simulink model "myExampleModel"  (R2026a)
settings: Solver=FixedStepDiscrete  StopTime=steps  FixedStep=1
model workspace (MAT data in the model file):
  net = dlnetwork
  net.any.Version = 6
  net.any.LayerGraph = nnet.cnn.LayerGraph
  net.any.LayerGraph.any.Version = 1
  net.any.LayerGraph.any.Layers(1) = nnet.cnn.layer.SequenceInputLayer
  net.any.LayerGraph.any.Layers(1).any.Version = 5
  net.any.LayerGraph.any.Layers(1).any.Name = 'sequenceinput'
  net.any.LayerGraph.any.Layers(1).any.InputSize = 5
  net.any.LayerGraph.any.Layers(1).any.Normalization.Version = 1
  net.any.LayerGraph.any.Layers(1).any.Normalization.Type = 'zscore'
  net.any.LayerGraph.any.Layers(1).any.Normalization.ImageSize = 5
  net.any.LayerGraph.any.Layers(1).any.Normalization.Mean = [0.711946004247; 0.753163225915; 0.731572433704; 0.711407042817; 0.753343332248]
  net.any.LayerGraph.any.Layers(1).any.Normalization.Std = [0.253594852887; 0.0795590152826; 0.271454001973; 0.250256363005; 0.0564169836974]
  net.any.LayerGraph.any.Layers(1).any.NormalizationDimension = 'auto'
  net.any.LayerGraph.any.Layers(1).any.MinLength = 1
  net.any.LayerGraph.any.Layers(1).any.SplitComplexInputs = 0
  net.any.LayerGraph.any.Layers(2) = nnet.cnn.layer.LSTMLayer
  net.any.LayerGraph.any.Layers(2).any.Version = 5
  net.any.LayerGraph.any.Layers(2).any.Name = 'lstm'
  net.any.LayerGraph.any.Layers(2).any.InputSize = 5
  net.any.LayerGraph.any.Layers(2).any.NumHiddenUnits = 32
  net.any.LayerGraph.any.Layers(2).any.ReturnSequence = 1
  net.any.LayerGraph.any.Layers(2).any.StateActivationFunction = 'tanh'
  net.any.LayerGraph.any.Layers(2).any.GateActivationFunction = 'sigmoid'
  net.any.LayerGraph.any.Layers(2).any.HasStateInputs = 0
  net.any.LayerGraph.any.Layers(2).any.HasStateOutputs = 0
  net.any.LayerGraph.any.Layers(2).any.InputWeights.Version = 2
  net.any.LayerGraph.any.Layers(2).any.InputWeights.Value = [0.158725649118 0.0836796313524 0.0394077338278 0.00389027385972 0.00940972659737 -0.159172236919 0.180239677429 0.0973209440708 -0.0486048273742 0.142829716206 0.0468379706144 -0.109037384391 ... (640 elements, 128x5)]
  net.any.LayerGraph.any.Layers(2).any.InputWeights.LearnRateFactor = 1
  net.any.LayerGraph.any.Layers(2).any.InputWeights.L2Factor = 1
  net.any.LayerGraph.any.Layers(2).any.InputWeights.Initializer.Version = 1
  net.any.LayerGraph.any.Layers(2).any.InputWeights.Initializer.Class = 'nnet.internal.cnn.layer.learnable.initializer.Glorot'
  net.any.LayerGraph.any.Layers(2).any.InputWeights.Initializer.ConstructorArguments = {2, 1}
  net.any.LayerGraph.any.Layers(2).any.RecurrentWeights.Version = 2
  net.any.LayerGraph.any.Layers(2).any.RecurrentWeights.Value = [-0.0278804842383 -0.025140536949 -0.0255219098181 -0.0234189406037 -0.0516594834626 -0.0393797829747 -0.0177398081869 -0.0392154678702 -0.105208314955 -0.100077986717 -0.0357415638864 0.0239775925875 ... (4096 elements, 128x32)]
  net.any.LayerGraph.any.Layers(2).any.RecurrentWeights.LearnRateFactor = 1
  net.any.LayerGraph.any.Layers(2).any.RecurrentWeights.L2Factor = 1
  net.any.LayerGraph.any.Layers(2).any.RecurrentWeights.Initializer.Version = 1
  net.any.LayerGraph.any.Layers(2).any.RecurrentWeights.Initializer.Class = 'nnet.internal.cnn.layer.learnable.initializer.Orthogonal'
  net.any.LayerGraph.any.Layers(2).any.RecurrentWeights.Initializer.ConstructorArguments = []
  net.any.LayerGraph.any.Layers(2).any.Bias.Version = 2
  net.any.LayerGraph.any.Layers(2).any.Bias.Value = [-0.0182774588466 0.0614794008434 0.0734638869762 -0.0580208562315 -0.0653121620417 0.113746903837 0.0700471177697 0.0615480169654 0.0146696139127 0.0178057868034 0.0246399398893 0.0890641435981 ... (128 elements, 128x1)]
  net.any.LayerGraph.any.Layers(2).any.Bias.LearnRateFactor = 1
  net.any.LayerGraph.any.Layers(2).any.Bias.L2Factor = 0
  net.any.LayerGraph.any.Layers(2).any.Bias.Initializer.Version = 1
  net.any.LayerGraph.any.Layers(2).any.Bias.Initializer.Class = 'nnet.internal.cnn.layer.learnable.initializer.UnitForgetGate'
  net.any.LayerGraph.any.Layers(2).any.Bias.Initializer.ConstructorArguments = {'LSTM'}
  net.any.LayerGraph.any.Layers(2).any.CellState.Value = [0; 0; 0; 0; 0; 0; 0; 0; 0; 0; 0; 0; 0; 0; 0; 0; 0; 0; 0; 0; 0; 0; 0; 0; 0; 0; 0; 0; 0; 0; 0; 0]
  net.any.LayerGraph.any.Layers(2).any.CellState.Remember = 1
  net.any.LayerGraph.any.Layers(2).any.HiddenState.Value = [0; 0; 0; 0; 0; 0; 0; 0; 0; 0; 0; 0; 0; 0; 0; 0; 0; 0; 0; 0; 0; 0; 0; 0; 0; 0; 0; 0; 0; 0; 0; 0]
  net.any.LayerGraph.any.Layers(2).any.HiddenState.Remember = 1
  net.any.LayerGraph.any.Layers(2).any.InitialCellState = [0; 0; 0; 0; 0; 0; 0; 0; 0; 0; 0; 0; 0; 0; 0; 0; 0; 0; 0; 0; 0; 0; 0; 0; 0; 0; 0; 0; 0; 0; 0; 0]
  net.any.LayerGraph.any.Layers(2).any.InitialHiddenState = [0; 0; 0; 0; 0; 0; 0; 0; 0; 0; 0; 0; 0; 0; 0; 0; 0; 0; 0; 0; 0; 0; 0; 0; 0; 0; 0; 0; 0; 0; 0; 0]
  net.any.LayerGraph.any.Layers(3) = nnet.cnn.layer.FullyConnectedLayer
  net.any.LayerGraph.any.Layers(3).any.Version = 5
  net.any.LayerGraph.any.Layers(3).any.Name = 'fc'
  net.any.LayerGraph.any.Layers(3).any.InputSize = []
  net.any.LayerGraph.any.Layers(3).any.OutputSize = 1
  net.any.LayerGraph.any.Layers(3).any.Weights.Version = 2
  net.any.LayerGraph.any.Layers(3).any.Weights.Value = [-0.0115323774517 -0.22575378418 0.0668845772743 0.308706641197 0.18884755671 0.224740937352 0.278032541275 0.305149555206 -0.0114221740514 -0.165821552277 -0.413473755121 -0.363296926022 -0.351468086243 0.283178627491 -0.0468922816217 -0.19526720047 0.115473456681 0.11662748456 -0.427064061165 0.384527653456 -0.253217667341 -0.318987667561 -0.351537317038 0.306988537312 -0.314961463213 0.122481673956 0.0571382455528 0.390641868114 0.372646659613 0.330578863621 -0.47236636281 0.24124994874]
  net.any.LayerGraph.any.Layers(3).any.Weights.LearnRateFactor = 1
  net.any.LayerGraph.any.Layers(3).any.Weights.L2Factor = 1
  net.any.LayerGraph.any.Layers(3).any.Weights.Initializer.Version = 1
  net.any.LayerGraph.any.Layers(3).any.Weights.Initializer.Class = 'nnet.internal.cnn.layer.learnable.initializer.Glorot'
  net.any.LayerGraph.any.Layers(3).any.Weights.Initializer.ConstructorArguments = {2, 1}
  net.any.LayerGraph.any.Layers(3).any.Bias.Version = 2
  net.any.LayerGraph.any.Layers(3).any.Bias.Value = -0.000715207715984
  net.any.LayerGraph.any.Layers(3).any.Bias.LearnRateFactor = 1
  net.any.LayerGraph.any.Layers(3).any.Bias.L2Factor = 0
  net.any.LayerGraph.any.Layers(3).any.Bias.Initializer.Version = 1
  net.any.LayerGraph.any.Layers(3).any.Bias.Initializer.Class = 'nnet.internal.cnn.layer.learnable.initializer.Zeros'
  net.any.LayerGraph.any.Layers(3).any.Bias.Initializer.ConstructorArguments = []
  net.any.LayerGraph.any.Layers(3).any.InputLearnables = {}
  net.any.LayerGraph.any.Layers(3).any.OutputLearnables = {}
  net.any.LayerGraph.any.Layers(3).any.OperationDimension = 'spatial-channel'
  net.any.LayerGraph.any.Layers(4) = nnet.cnn.layer.InverseNormalizationLayer
  net.any.LayerGraph.any.Layers(4).Name = 'inversenorm'
  net.any.LayerGraph.any.Layers(4).Normalization = 'zscore'
  net.any.LayerGraph.any.Layers(4).OperationDimension = 'channel'
  net.any.LayerGraph.any.Layers(4).Mean = 0.633833984011
  net.any.LayerGraph.any.Layers(4).StandardDeviation = 0.340294791967
  net.any.LayerGraph.any.Connections = table
  net.any.LayerGraph.any.Connections.data = {{'sequenceinput'; 'lstm'; 'fc'}, {'lstm'; 'fc'; 'inversenorm'}}
  net.any.LayerGraph.any.Connections.ndims = 2
  net.any.LayerGraph.any.Connections.nrows = 3
  net.any.LayerGraph.any.Connections.nvars = 2
  net.any.LayerGraph.any.Connections.varnames = {'Source', 'Destination'}
  net.any.LayerGraph.any.Connections.props.CustomProps = struct()
  net.any.LayerGraph.any.Connections.props.VariableCustomProps = struct()
  net.any.LayerGraph.any.Connections.props.versionSavedFrom = 5
  net.any.LayerGraph.any.Connections.props.minCompatibleVersion = 1
  net.any.LayerGraph.any.Connections.props.incompatibilityMsg = ''
  net.any.LayerGraph.any.Connections.props.VersionSavedFrom = 5
  net.any.LayerGraph.any.Connections.props.useVariableNamesOriginal = 0
  net.any.LayerGraph.any.Connections.props.useVariableNames2048 = 0
  net.any.LayerGraph.any.Connections.props.useDimensionNamesOriginal = 0
  net.any.LayerGraph.any.Connections.props.useDimensionNames2048 = 0
  net.any.LayerGraph.any.Connections.props.Description = ''
  net.any.LayerGraph.any.Connections.props.VariableNamesOriginal = {}
  net.any.LayerGraph.any.Connections.props.VariableNames2048 = {}
  net.any.LayerGraph.any.Connections.props.DimensionNames = {'Row', 'Variables'}
  net.any.LayerGraph.any.Connections.props.DimensionNamesOriginal = {}
  net.any.LayerGraph.any.Connections.props.DimensionNames2048 = {}
  net.any.LayerGraph.any.Connections.props.UserData = []
  net.any.LayerGraph.any.Connections.props.VariableDescriptions = {}
  net.any.LayerGraph.any.Connections.props.VariableUnits = {}
  net.any.LayerGraph.any.Connections.props.VariableContinuity = {}
  net.any.Initialized = 1
  net.any.SerializedQuantizationInfo.version = 1
  net.any.SerializedQuantizationInfo.data = containers.Map
  net.any.SerializedQuantizationInfo.data.serialization.keys = {}
  net.any.SerializedQuantizationInfo.data.serialization.values = {}
  net.any.SerializedQuantizationInfo.data.serialization.uniformity = 0
  net.any.SerializedQuantizationInfo.data.serialization.keyType = 'char'
  net.any.SerializedQuantizationInfo.data.serialization.valueType = 'any'
  net.any.ExampleInputs = {}
  net.any.OutputNames = {'inversenorm'}
  net.any.ExternalOutputNames = []
  net.any.ExternalInputNames = []
  net.any.RetainCustomInputNames = 1
  net.any.RetainCustomOutputNames = 1
libraries: dlinputlayernormlib x2, dlconvfclib x1, dlsequencelib x1
settings Model: Creator=jianghaw  LastModifiedBy=wenzheli
settings SFSimCC: SimTargetLang=C++
settings RTWCC: SystemTargetFile=ert.tlc  Description=Embedded Coder
settings ERTTargetCC: GenerateSampleERTMain=on

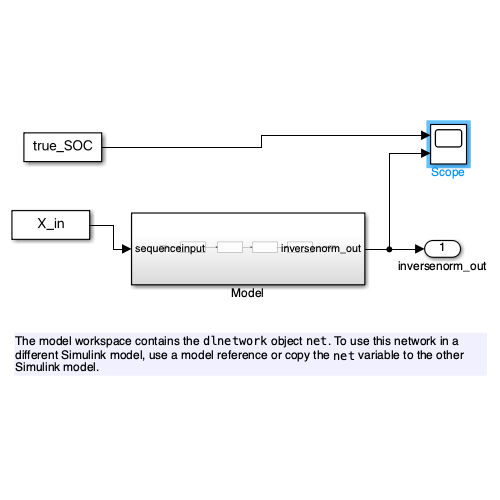
[thumbnail: Simulink's stored preview of the top-level diagram]
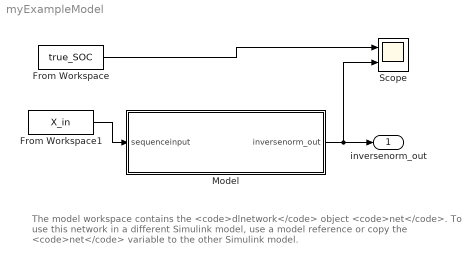
== system myExampleModel ==
  note: The model workspace contains the <code>dlnetwork</code> object <code>net</code>. To use this network in a different Simulink model, use a model reference or copy the <code>net</code> variable to the other Simulink model.
  From Workspace : FromWorkspace  VariableName=true_SOC
  From Workspace1 : FromWorkspace  VariableName=X_in
  Model : Subsystem
  Scope : Scope  NumInputPorts=2
      settings: ActiveDisplayYMinimum=0.10294478759169581  ActiveDisplayYMaximum=1.1551280356943607
  inversenorm_out : Outport
  wires:
  Model/1(inversenorm_out) -> Scope/2, inversenorm_out/1
  From Workspace1/1 -> Model/1(sequenceinput)
  From Workspace/1 -> Scope/1

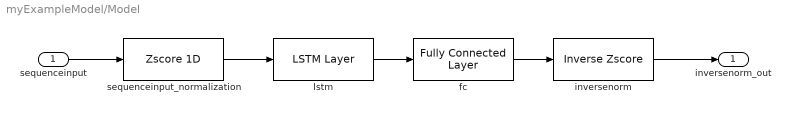
== system myExampleModel/Model ==
  sequenceinput : Inport  PortDimensions="[5  1]"
  fc : dlconvfclib/Fully Connected Layer  Layer=net.Layers(3)  OutMin=[]  OutMax=[]  WeightsDataTypeStr=Inherit: Inherit via back propagation  WeightsMin=[]  WeightsMax=[]  BiasDataTypeStr=Inherit: Inherit via back propagation  BiasMin=[]  BiasMax=[]  AccumMin=[]  AccumMax=[]  InternalRndMeth=Floor  InternalSaturateOnIntegerOverflow=off  SampleTime=-1
      settings: DataFormat=CT
  inversenorm : dlinputlayernormlib/Inverse Zscore  Layer=net.Layers(4)  OutMin=[]  OutMax=[]  MeanDataTypeStr=Inherit: Inherit via back propagation  MeanMin=[]  MeanMax=[]  StandardDeviationDataTypeStr=Inherit: Inherit via back propagation  StandardDeviationMin=[]  StandardDeviationMax=[]  InternalRndMeth=Floor  InternalSaturateOnIntegerOverflow=off  SampleTime=-1
      settings: DataFormat=CT
  lstm : dlsequencelib/LSTM Layer  Layer=net.Layers(2)  Stateful=on  ApproximationMethod=None  OutMin=[]  OutMax=[]  InputWeightsDataTypeStr=Inherit: Inherit via back propagation  InputWeightsMin=[]  InputWeightsMax=[]  RecurrentWeightsDataTypeStr=Inherit: Inherit via back propagation  RecurrentWeightsMin=[]  RecurrentWeightsMax=[]  BiasDataTypeStr=Inherit: Inherit via back propagation  BiasMin=[]  BiasMax=[]  InitialCellStateDataTypeStr=Inherit: Inherit via back propagation  InitialCellStateMin=[]  InitialCellStateMax=[]  CellStateMin=[]  CellStateMax=[]  InitialHiddenStateDataTypeStr=Inherit: Inherit via back propagation  InitialHiddenStateMin=[]  InitialHiddenStateMax=[]  HiddenStateMin=[]  HiddenStateMax=[]  InputWeightsMatrixMultiplyOutMin=[]  InputWeightsMatrixMultiplyOutMax=[]  RecurrentWeightsMatrixMultiplyOutMin=[]  RecurrentWeightsMatrixMultiplyOutMax=[]  LinearGateAddOutMin=[]  LinearGateAddOutMax=[]  CellStateProductOutMin=[]  CellStateProductOutMax=[]  SampleTime=-1
      settings: DataFormat=CT
  sequenceinput_normalization : dlinputlayernormlib/Zscore 1D  Layer=net.Layers(1)  OutMin=[]  OutMax=[]  MeanDataTypeStr=Inherit: Inherit via back propagation  MeanMin=[]  MeanMax=[]  StandardDeviationDataTypeStr=Inherit: Inherit via back propagation  StandardDeviationMin=[]  StandardDeviationMax=[]  AccumMin=[]  AccumMax=[]  InternalRndMeth=Floor  InternalSaturateOnIntegerOverflow=off  SampleTime=-1
      settings: DataFormat=CT
  inversenorm_out : Outport
  wires:
  sequenceinput_normalization/1 -> lstm/1
  lstm/1 -> fc/1
  fc/1 -> inversenorm/1
  inversenorm/1 -> inversenorm_out/1
  sequenceinput/1 -> sequenceinput_normalization/1
